simulink model "task3_alternate_try"  (R2023b)
settings: Solver=FixedStepDiscrete  StartTime=0.0  StopTime=15  FixedStep=5e-5  RelTol=1e-3
PreLoadFcn:
  | Simulink.defineIntEnumType('windowCommand', {'Off','Speed1','Speed2','Speed3'},[0,1,2,3])
undefined symbols (not defined in the file): windowCommand
libraries: simulink x5, slpidlib x1
settings Model: Creator=kz1nz0  LastModifiedBy=User

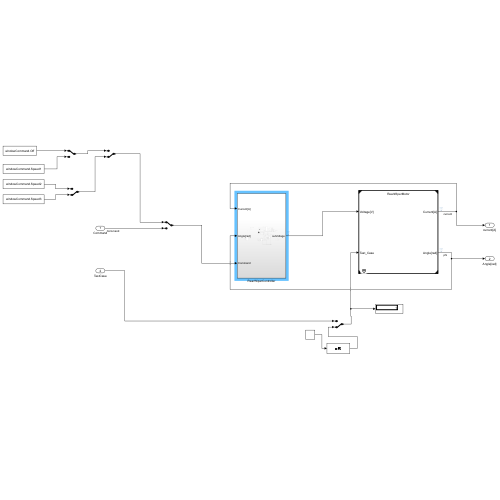
[thumbnail: Simulink's stored preview of the top-level diagram]
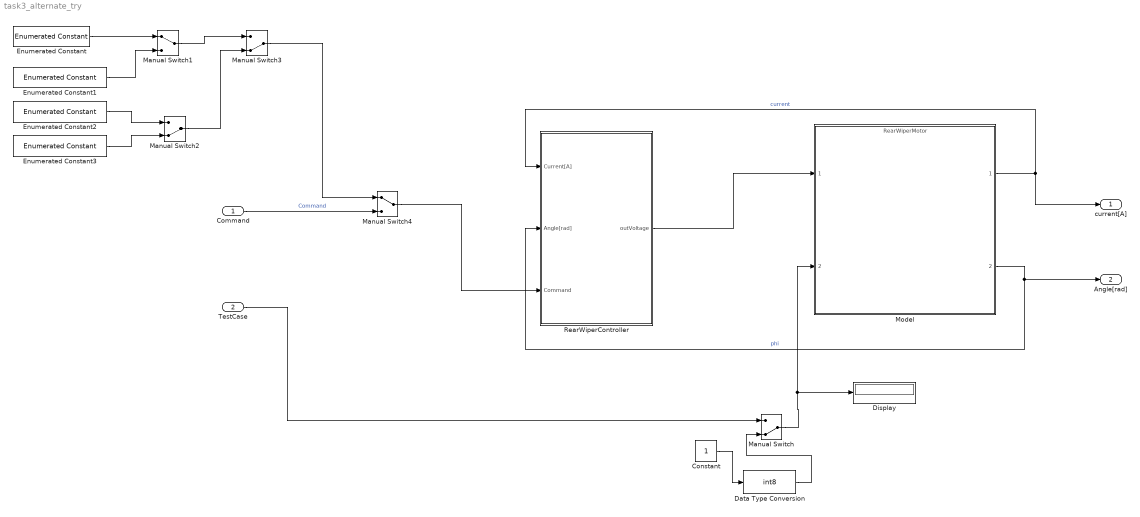
== system task3_alternate_try ==
  Command : Inport  OutDataTypeStr=Enum: windowCommand
  TestCase : Inport  Port=2  OutDataTypeStr=int8
  Constant : Constant
  Data Type Conversion : DataTypeConversion  OutDataTypeStr=int8  SaturateOnIntegerOverflow=off  RndMeth=Floor
  Display : Display
  Enumerated Constant : simulink/Sources/Enumerated Constant  OutDataTypeStr=Enum: windowCommand  Value=windowCommand.Off  SampleTime=inf
  Enumerated Constant1 : simulink/Sources/Enumerated Constant  OutDataTypeStr=Enum: windowCommand  Value=windowCommand.Speed1  SampleTime=inf
  Enumerated Constant2 : simulink/Sources/Enumerated Constant  OutDataTypeStr=Enum: windowCommand  Value=windowCommand.Speed2  SampleTime=inf
  Enumerated Constant3 : simulink/Sources/Enumerated Constant  OutDataTypeStr=Enum: windowCommand  Value=windowCommand.Speed3  SampleTime=inf
  Manual Switch : ManualSwitch  CurrentSetting=0
  Manual Switch1 : ManualSwitch
  Manual Switch2 : ManualSwitch  CurrentSetting=0
  Manual Switch3 : ManualSwitch  CurrentSetting=0
  Manual Switch4 : ManualSwitch
  Model : ModelReference  ModelNameDialog=RearWiperMotor.slxp  ModelReferenceVersion=19.15  CopyOfModelProtected=on
  RearWiperController : Subsystem
  current[A] : Outport
  Angle[rad] : Outport  Port=2
  wires:
  Command/1 -> Manual Switch4/2  "Command"
  TestCase/1 -> Manual Switch/1
  Model/1 -> current[A]/1, RearWiperController/1(Current[A])  "current"
  Model/2 -> RearWiperController/2(Angle[rad]), Angle[rad]/1  "phi"
  RearWiperController/1(outVoltage) -> Model/1
  Constant/1 -> Data Type Conversion/1
  Data Type Conversion/1 -> Manual Switch/2
  Manual Switch/1 -> Display/1, Model/2
  Enumerated Constant/1 -> Manual Switch1/1
  Manual Switch1/1 -> Manual Switch3/1
  Enumerated Constant3/1 -> Manual Switch2/2
  Manual Switch2/1 -> Manual Switch3/2
  Enumerated Constant1/1 -> Manual Switch1/2
  Enumerated Constant2/1 -> Manual Switch2/1
  Manual Switch3/1 -> Manual Switch4/1
  Manual Switch4/1 -> RearWiperController/3(Command)

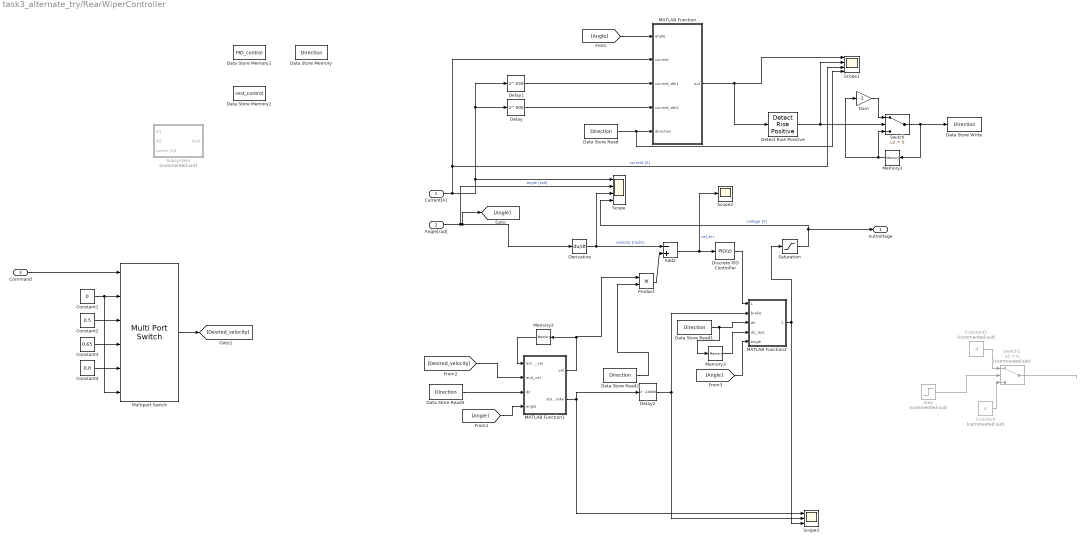
== system task3_alternate_try/RearWiperController ==
  Current[A] : Inport
  Angle[rad] : Inport  Port=2
  Command : Inport  Port=3  OutDataTypeStr=Enum: windowCommand
  Add2 : Sum  Inputs=-+
  Constant : Constant  Commented=on  Value=4
  Constant1 : Constant  Value=0
  Constant2 : Constant  Value=0.5
  Constant3 : Constant  Value=0.65
  Constant4 : Constant  Value=0.8
  Constant5 : Constant  Commented=on  Value=-4
  Data Store Memory : DataStoreMemory  DataStoreName=Direction  WriteAfterWriteMsg=warning  InitialValue=1  ShowAdditionalParam=off
  Data Store Memory1 : DataStoreMemory  DataStoreName=PID_control  WriteAfterWriteMsg=warning  InitialValue=1  ShowAdditionalParam=off
  Data Store Memory2 : DataStoreMemory  DataStoreName=rest_control  WriteAfterWriteMsg=warning  InitialValue=4  ShowAdditionalParam=off
  Data Store Read{,1..3} (4 alike) : DataStoreRead  DataStoreName=Direction  IndexOptions=Index vector (dialog)  Indices=1  OutputSizes=1
  Data Store Write : DataStoreWrite  DataStoreName=Direction  IndexOptions=Index vector (dialog)  Indices=1  OutputSizes=1
  Delay : Delay  DelayLength=500
  Delay1 : Delay  DelayLength=250
  Delay2 : Delay  DelayLength=10000
  Derivative : Derivative
  Detect Rise Positive : simulink/Logic and Bit Operations/Detect Rise Positive  vinit=0  OutDataTypeStr=boolean
  Discrete PID Controller : slpidlib/PID Controller  Controller=PID  Form=Parallel  TimeDomain=Discrete-time  UseExternalTs=off  SampleTime=-1  IntegratorMethod=Forward Euler  FilterMethod=Forward Euler  ControllerParametersSource=internal  P=70  I=40  UseKiTs=off  D=5  N=100  UseFilter=on  TunerSelectOption=Frequency Response Based  InitialConditionSource=internal  InitialConditionForIntegrator=0  InitialConditionForFilter=0  DifferentiatorICPrevScaledInput=0  ExternalReset=none  TrackingMode=off  Kt=1  LimitOutput=off  SatLimitsSource=internal  UpperSaturationLimit=inf  LowerSaturationLimit=-inf  LinearizeAsGain=off  AntiWindupMode=none  Kb=1  LimitIntegrator=off  UpperIntegratorSaturationLimit=inf  LowerIntegratorSaturationLimit=-inf  POutMin=[]  POutMax=[]  IOutMin=[]  IOutMax=[]  DOutMin=[]  DOutMax=[]  NOutMin=[]  NOutMax=[]  SumOutMin=[]  SumOutMax=[]  SaturationOutMin=[]  SaturationOutMax=[]  PParamMin=[]  PParamMax=[]  IParamMin=[]  IParamMax=[]  DParamMin=[]  DParamMax=[]  NParamMin=[]  NParamMax=[]  KbParamMin=[]  KbParamMax=[]  KtParamMin=[]  KtParamMax=[]  KbOutMin=[]  KbOutMax=[]  KtOutMin=[]  KtOutMax=[]  IntegratorOutMin=[]  IntegratorOutMax=[]  FilterOutMin=[]  FilterOutMax=[]  SumI1OutMin=[]  SumI1OutMax=[]  SumI2OutMin=[]  SumI2OutMax=[]  SumI3OutMin=[]  SumI3OutMax=[]  SumI4OutMin=[]  SumI4OutMax=[]  SumDOutMin=[]  SumDOutMax=[]  DifferentiatorOutMin=[]  DifferentiatorOutMax=[]  FilterDiffOutCoefMin=[]  FilterDiffOutCoefMax=[]  ReciprocalOutMin=[]  ReciprocalOutMax=[]  SumDenOutMin=[]  SumDenOutMax=[]  SumNumOutMin=[]  SumNumOutMax=[]  DivideOutMin=[]  DivideOutMax=[]  UdiffTsProdOutMin=[]  UdiffTsProdOutMax=[]  NTsProdOutMin=[]  NTsProdOutMax=[]  UintegralTsProdOutMin=[]  UintegralTsProdOutMax=[]  UngainTsProdOutMin=[]  UngainTsProdOutMax=[]  ClampingZeroOutDataTypeStr=Inherit: Inherit via back propagation  ClampingZeroOutMin=[]  ClampingZeroOutMax=[]  FilterDenConstantOutDataTypeStr=Inherit: Inherit via back propagation  FilterDenConstantOutMin=[]  FilterDenConstantOutMax=[]  PCopyOutDataTypeStr=Inherit: Inherit via back propagation  PCopyOutMin=[]  PCopyOutMax=[]  NCopyOutDataTypeStr=Inherit: Inherit via back propagation  NCopyOutMin=[]  NCopyOutMax=[]  IntegratorContinuousStateAttributes=''  IntegratorStateMustResolveToSignalObject=off  IntegratorRTWStateStorageClass=Auto  FilterContinuousStateAttributes=''  FilterStateMustResolveToSignalObject=off  FilterRTWStateStorageClass=Auto  ParallelPVariant=InternalParameters  IdealPVariant=Disabled  IVariant=InternalParameters  DVariant=InternalParameters  IntegratorVariant=Discrete  SatVariant=Disabled  AWVariant=Passthrough  PCopyVariant=Disabled  TRVariant=Disabled  FdbkBlocksVariant=Forward  IdealPFdbkVariant=Disabled  SatFdbkVariant=Disabled  DerivativeFilterVariant=ForwardEulerFilter  NVariant=InternalParameters  NCopyVariant=Disabled  FilterICVariant=InternalICsFilter  IntegratorICVariant=InternalICs  ExternalResetVariant=Disabled  TRSumVariant=Passthrough  SumFdbkVariant=Disabled  SumVariant=Sum_PID  TsampFilterVariant=InternalTs  TsampNgainVariant=Passthrough  TsampIntegralVariant=Disabled_SignalSpec  ExternalSaturationOutDataTypeStr=Inherit: Same as second input
      settings: LibrarySourceBlock=simulink/Discrete/Discrete PID Controller
  Gain : Gain  Gain=-1
  MATLAB Function : MATLAB Function  TreatAsAtomicUnit=on
  MATLAB Function1 : MATLAB Function  TreatAsAtomicUnit=on
  MATLAB Function2 : MATLAB Function  TreatAsAtomicUnit=on
  Memory1 : Memory  InitialCondition=1
  Memory2 : Memory
  Memory3 : Memory  InitialCondition=1
  Multiport Switch : MultiPortSwitch  DataPortOrder=Specify indices  DataPortIndices={windowCommand.Off, windowCommand.Speed1, windowCommand.Speed2, windowCommand.Speed3}  DataPortForDefault=Additional data port  SaturateOnIntegerOverflow=off  InputSameDT=off
  Product : Product
  Saturation : Saturate  UpperLimit=12  LowerLimit=-12
  Scope : Scope  NumInputPorts=4
  Scope1 : Scope  NumInputPorts=4
  Scope2 : Scope
  Scope3 : Scope  NumInputPorts=3
  Step : Step  Commented=on  Time=5  SampleTime=0
  Subsystem : Subsystem  Commented=on
  Switch : Switch  Criteria=u2 > Threshold  SaturateOnIntegerOverflow=off  InputSameDT=off
  Switch1 : Switch  Commented=on  Criteria=u2 > Threshold  SaturateOnIntegerOverflow=off  InputSameDT=off
  outVoltage : Outport
  wires:
  Current[A]/1 -> Delay/1, Delay1/1, Scope/1, Scope1/3, MATLAB Function/2(current)  "current [A]"
  Angle[rad]/1 -> Derivative/1, [Angle], Scope/2  "angle [rad]"
  Multiport Switch/1 -> [Desired_velocity]
  Constant2/1 -> Multiport Switch/3
  Constant3/1 -> Multiport Switch/4
  Constant4/1 -> Multiport Switch/5
  Constant1/1 -> Multiport Switch/6, Multiport Switch/2
  Saturation/1 -> outVoltage/1, Scope/4  "voltage [V]"
  Derivative/1 -> Scope/3, Add2/1  "velocity [rad/s]"
  Command/1 -> Multiport Switch/1
  Detect Rise Positive/1 -> Scope1/2, Switch/2
  Switch/1 -> Memory1/1, Data Store Write/1
  Memory1/1 -> Gain/1, Switch/3
  Gain/1 -> Switch/1
  Delay1/1 -> MATLAB Function/3(current_del1)
  Delay/1 -> MATLAB Function/4(current_del2)
  [Angle] -> MATLAB Function/1(angle)
  Data Store Read/1 -> Scope1/4, MATLAB Function/5(direction)
  MATLAB Function/1(out) -> Scope1/1, Detect Rise Positive/1
  Product/1 -> Add2/2
  Data Store Read2/1 -> Product/2
  Add2/1 -> Scope2/1, Discrete PID Controller/1  "vel_err"
  Discrete PID Controller/1 -> MATLAB Function2/1(PID_out)
  MATLAB Function1/1(vel) -> Product/1, Memory2/1
  Memory2/1 -> MATLAB Function1/1(actual_vel)
  [Angle] -> MATLAB Function1/4(angle)
  Data Store Read3/1 -> MATLAB Function1/3(dir)
  MATLAB Function2/1(outVoltage) -> Scope3/3, Saturation/1
  Data Store Read1/1 -> Memory3/1, MATLAB Function2/3(dir)
  [Angle] -> MATLAB Function2/5(angle)
  [Desired_velocity] -> MATLAB Function1/2(end_vel)
  Constant5/1 -> Switch1/1
  Constant/1 -> Switch1/3
  Switch1/1 -> ?
  Step/1 -> Switch1/2
  MATLAB Function1/2(start_brake) -> Scope3/1, Delay2/1
  Delay2/1 -> MATLAB Function2/2(brake), Scope3/2
  Memory3/1 -> MATLAB Function2/4(dir_last)

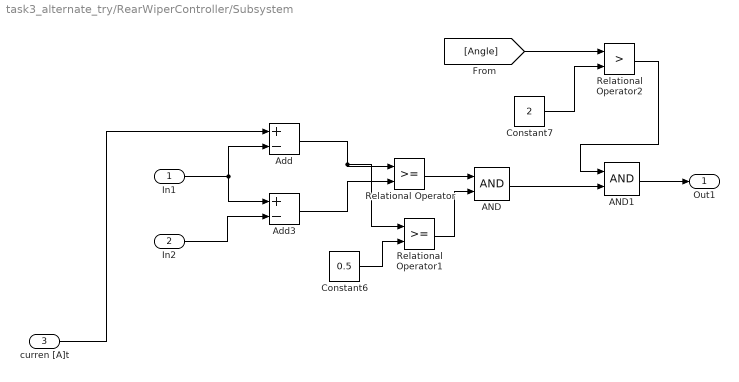
== system task3_alternate_try/RearWiperController/Subsystem ==
  In1 : Inport
  In2 : Inport  Port=2
  curren [A]t : Inport  Port=3
  AND : Logic  AllPortsSameDT=off  OutDataTypeStr=boolean
  AND1 : Logic  AllPortsSameDT=off  OutDataTypeStr=boolean
  Add : Sum  Inputs=+-
  Add3 : Sum  Inputs=+-
  Constant6 : Constant  Value=0.5
  Constant7 : Constant  Value=2
  Relational Operator : RelationalOperator  OutDataTypeStr=boolean  RndMeth=Simplest  InputSameDT=off
  Relational Operator1 : RelationalOperator  OutDataTypeStr=boolean  RndMeth=Simplest  InputSameDT=off
  Relational Operator2 : RelationalOperator  Operator=>  OutDataTypeStr=boolean  RndMeth=Simplest  InputSameDT=off
  Out1 : Outport
  wires:
  AND/1 -> AND1/2
  Relational Operator/1 -> AND/1
  curren [A]t/1 -> Add/1
  [Angle] -> Relational Operator2/1
  Relational Operator2/1 -> AND1/1
  Add3/1 -> Relational Operator/2
  Constant6/1 -> Relational Operator1/2
  In1/1 -> Add3/1, Add/2
  Add/1 -> Relational Operator1/1, Relational Operator/1
  Relational Operator1/1 -> AND/2
  Constant7/1 -> Relational Operator2/2
  AND1/1 -> Out1/1
  In2/1 -> Add3/2

== matlab function task3_alternate_try/RearWiperController/MATLAB Function1 ==
  data: actual_vel input; vel output; end_vel input; dir input; angle input; start_brake output
function [vel, start_brake] = desired_velocity(actual_vel, end_vel, dir, angle)


angle_tresh_pos = 2;    % [rad]
angle_tresh_neg = 0.7;    % [rad]
step = 5e-5;            % [rad/s]

step2 = 3e-5;           % [rad/s]

rest_vel = 0.2;         % [rad/s]

if (dir == 1 && angle > angle_tresh_pos) || (dir == -1 && angle < angle_tresh_neg)
    
    if actual_vel > rest_vel
        vel = actual_vel - step2;
    else
        vel = rest_vel;
    end

    start_brake = 1;

else

    if actual_vel < end_vel
        vel = actual_vel + step;
    else
        vel = end_vel;
    end

    start_brake = 0;
end

== matlab function task3_alternate_try/RearWiperController/MATLAB Function ==
  data: angle input; current input; out output; current_del1 input; current_del2 input; direction input
function out = change_direction(angle, current, current_del1, current_del2, direction)


curr_diff_tresh = 0.5; % [A]
angle_tresh_pos = 2; % [rad]
angle_tresh_neg = 1; % [rad]

% direction = -1  -> obrót w lewo (ujemne napięcie)
% direction = 1  -> obrót w prawo (dodatnie napięcie)

if(direction == -1)
    out = ((current_del1 - current) >= (current_del2 - current_del1) && (current_del1 - current) > curr_diff_tresh) && angle < angle_tresh_neg;

elseif(direction == 1)
    out = ((current - current_del1) >= (current_del1 - current_del2) && (current - current_del1) > curr_diff_tresh) && angle > angle_tresh_pos;

else
    out = true;
end

== matlab function task3_alternate_try/RearWiperController/MATLAB Function2 ==
  data: PID_out input; brake input; outVoltage output; dir input; dir_last input; angle input
function outVoltage =  fcn(PID_out, brake, dir, dir_last, angle)


rest_voltage = 4;       %[V]

angle_tresh_pos = 2;    % [rad]
angle_tresh_neg = 1;    % [rad]


step = 5e-5;            % [rad/s]

step2 = 2e-5;            % [rad/s]



if brake

    outVoltage = rest_voltage;

else

    outVoltage = PID_out;

end

%outVoltage = PID_out;
